simulink model "COMPARISON_bf"  (Simulink 9.2)
settings: Solver=ode45  StartTime=0.0  StopTime=5  RelTol=1e-3  EnableMultiTasking=on
undefined symbols (not defined in the file or in its folder): kp1, kp2, kv1, kv2
settings Model: Creator=japerez  LastModifiedBy=a.brugnoli
settings DataIOCC: SignalLoggingSaveFormat=Dataset
settings DebuggingCC: UnderspecifiedInitializationDetection=Simplified  MergeDetectMultiDrivingBlocksExec=error  SolverPrmCheckMsg=warning  FcnCallInpInsideContextMsg=error  AllowSymbolicDim=off  StateNameClashWarn=none
settings GRTTargetCC: CombineOutputUpdateFcns=on  GRTInterface=off
settings ConfigComp: CovSFcnEnable=off

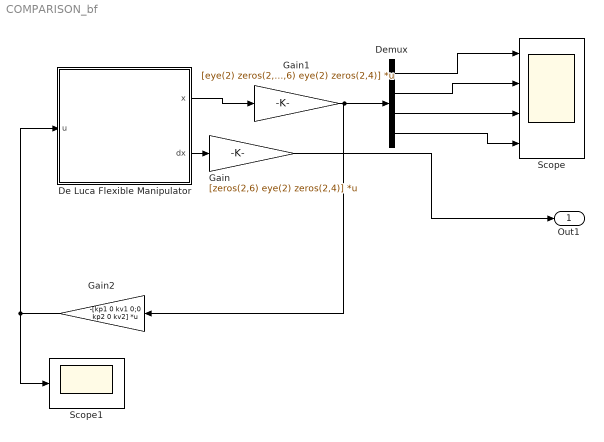
== system COMPARISON_bf ==
  De Luca Flexible Manipulator : Subsystem
  Demux : Demux
  Gain : Gain  Gain=[zeros(2,6) eye(2) zeros(2,4)]  Multiplication=Matrix(K*u) (u vector)
  Gain1 : Gain  Gain=[eye(2) zeros(2,10); zeros(2,6) eye(2) zeros(2,4)]  Multiplication=Matrix(K*u) (u vector)
  Gain2 : Gain  Gain="-[kp1 0 kv1 0;0  kp2 0  kv2]"  Multiplication=Matrix(K*u) (u vector)
  Scope : Scope  NumInputPorts=4
  Scope1 : Scope
  Out1 : Outport
  wires:
  Gain2/1 -> De Luca Flexible Manipulator/1(u), Scope1/1
  De Luca Flexible Manipulator/1(x) -> Gain1/1
  De Luca Flexible Manipulator/2(dx) -> Gain/1
  Gain/1 -> Out1/1
  Gain1/1 -> Gain2/1, Demux/1
  Demux/1 -> Scope/1
  Demux/2 -> Scope/2
  Demux/3 -> Scope/3
  Demux/4 -> Scope/4

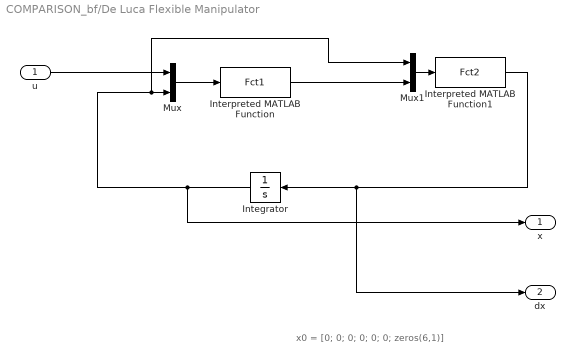
== system COMPARISON_bf/De Luca Flexible Manipulator ==
  note: x0 = [0; 0; 0; 0; 0; 0; zeros(6,1)]
  u : Inport  PortDimensions=2
  Integrator : Integrator  InitialCondition=[0; 10*pi/180; 0; 0; 0; 0; zeros(6,1)]
  Interpreted MATLAB Function : MATLABFcn  MATLABFcn=Fct1  OutputDimensions=12
  Interpreted MATLAB Function1 : MATLABFcn  MATLABFcn=Fct2  OutputDimensions=12
  Mux : Mux  Inputs=[2 12]
  Mux1 : Mux  Inputs=[12 12]
  x : Outport  PortDimensions=12
  dx : Outport  Port=2  PortDimensions=12
  wires:
  u/1 -> Mux/1
  Interpreted MATLAB Function1/1 -> dx/1, Integrator/1
  Mux/1 -> Interpreted MATLAB Function/1
  Interpreted MATLAB Function/1 -> Mux1/2
  Integrator/1 -> x/1, Mux1/1, Mux/2
  Mux1/1 -> Interpreted MATLAB Function1/1
